simulink model "Golf_Lin_Optimale"  (R2019a)
settings: Solver=VariableStepAuto  StartTime=0.0  StopTime=4000  RelTol=1e-3
values from neighbouring files (symbols this model uses):
  A_sys = Alf(idx_states, idx_states)    [mainProjetCADV_2a.m]
  Ar = [-3/taero, 0 ... (first row only)    [mainProjetCADV_2a.m]
  B_sys = Blf(idx_states, idx_inputs)    [mainProjetCADV_2a.m]
  Br = [3/taero, 0 ... (first row only)    [mainProjetCADV_2a.m]
  C_sys = [1,  0, 0, 0 ... (first row only)    [mainProjetCADV_2a.m]
  Cr = eye(2)    [mainProjetCADV_2a.m]
  D_sys = zeros(4,2)    [mainProjetCADV_2a.m]
  DEG2RAD = pi/180.    (= 0.0174532925199)    [mainProjetCADV_2a.m]    (also in utAcDynamicsFunction.m; utConstantAeroCoeff.m)
  Dpf = K_aug * [Nx; Nxr] + Nu    [mainProjetCADV_2a.m]
  Dr = zeros(2,2)    [mainProjetCADV_2a.m]
  Kr = K_aug(:, 5:6)    [mainProjetCADV_2a.m]
  KTS2MS = 1852 / 3600    (= 0.514444444444)    [mainProjetCADV_2a.m]    (also in utAcDynamicsFunction.m)
  Kx = K_aug(:, 1:4)    [mainProjetCADV_2a.m]
  RAD2DEG = 180/pi    (= 57.2957795131)    [mainProjetCADV_2a.m]    (also in utAcDynamicsFunction.m)
settings Model: Creator=ulyss  LastModifiedBy=mariu

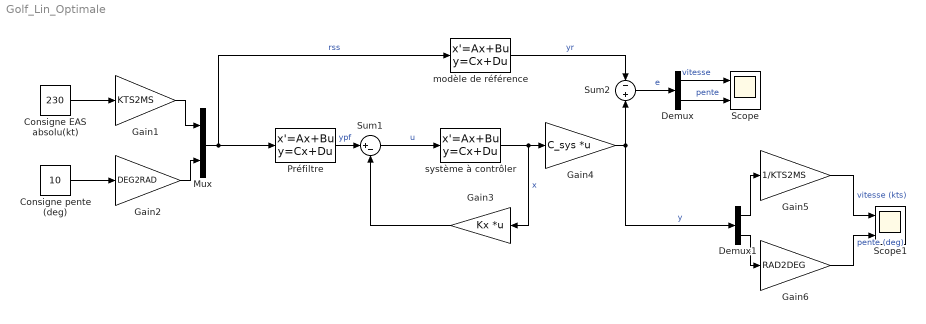
== system Golf_Lin_Optimale ==
  Consigne EAS absolu(kt) : Constant  Value=230
  Consigne pente (deg) : Constant  Value=10
  Demux : Demux  Outputs=2
  Demux1 : Demux  Outputs=2
  Gain1 : Gain  Gain=KTS2MS
  Gain2 : Gain  Gain=DEG2RAD
  Gain3 : Gain  Gain=Kx  Multiplication=Matrix(K*u) (u vector)
  Gain4 : Gain  Gain=C_sys  Multiplication=Matrix(K*u) (u vector)
  Gain5 : Gain  Gain=1/KTS2MS
  Gain6 : Gain  Gain=RAD2DEG
  Mux : Mux  Inputs=2
  Préfiltre : StateSpace  A=Ar  B=Br  C=-Kr  D=Dpf  InitialCondition=0
  Scope : Scope  NumInputPorts=2
  Scope1 : Scope  NumInputPorts=2
  Sum1 : Sum  Inputs=|+-
  Sum2 : Sum  Inputs=-|+
  modèle de référence : StateSpace  A=Ar  B=Br  C=Cr  D=Dr  InitialCondition="[260*KTS2MS,  -5*DEG2RAD]"
  système à contrôler : StateSpace  A=A_sys  B=B_sys  C=eye(4)  D=D_sys  InitialCondition=[260*KTS2MS, 0, -5*DEG2RAD, 0]
  wires:
  Consigne EAS absolu(kt)/1 -> Gain1/1
  Gain1/1 -> Mux/1
  Consigne pente (deg)/1 -> Gain2/1
  Gain2/1 -> Mux/2
  Mux/1 -> Préfiltre/1, modèle de référence/1  "rss"
  Préfiltre/1 -> Sum1/1  "ypf"
  système à contrôler/1 -> Gain4/1, Gain3/1  "x"
  Sum2/1 -> Demux/1  "e"
  Gain3/1 -> Sum1/2
  Sum1/1 -> système à contrôler/1  "u"
  Demux/1 -> Scope/1  "vitesse"
  Demux/2 -> Scope/2  "pente"
  modèle de référence/1 -> Sum2/1  "yr"
  Demux1/2 -> Gain6/1
  Gain4/1 -> Demux1/1, Sum2/2  "y"
  Demux1/1 -> Gain5/1
  Gain5/1 -> Scope1/1  "vitesse (kts)"
  Gain6/1 -> Scope1/2  "pente (deg)"
